simulink model "pointavg"  (R2024a)
settings: Solver=VariableStepDiscrete  StartTime=0.0  StopTime=65  RelTol=1e-3
settings Model: Creator=bag66  LastModifiedBy=bag66

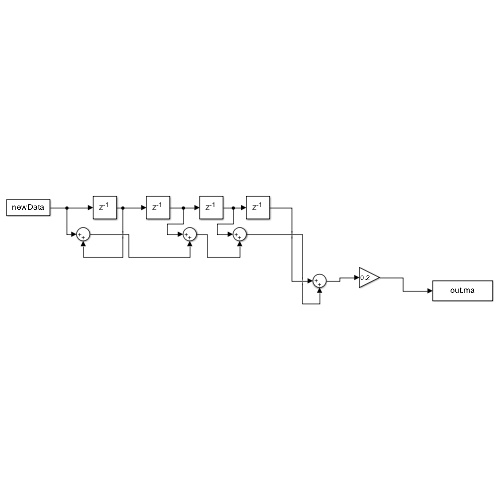
[thumbnail: Simulink's stored preview of the top-level diagram]
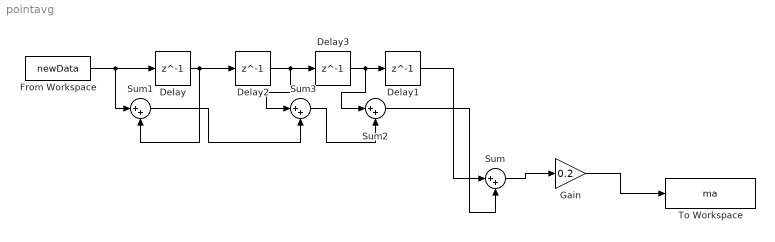
== system pointavg ==
  Delay{,1..3} (4 alike) : Delay  DelayLength=1  InitialCondition=0  SampleTime=1
  From Workspace : FromWorkspace  VariableName=newData  SampleTime=1
  Gain : Gain  Gain=0.2
  Sum{,1..3} (4 alike) : Sum  Inputs=|++
  To Workspace : ToWorkspace  VariableName=ma  SampleTime=1
      settings: Save2DSignal=2-D array (concatenate along first dimension)
  wires:
  From Workspace/1 -> Sum1/1, Delay/1
  Delay/1 -> Delay2/1, Sum1/2
  Delay2/1 -> Sum3/1, Delay3/1
  Delay3/1 -> Sum2/1, Delay1/1
  Delay1/1 -> Sum/1
  Sum3/1 -> Sum2/2
  Sum2/1 -> Sum/2
  Sum/1 -> Gain/1
  Gain/1 -> To Workspace/1
  Sum1/1 -> Sum3/2
